simulink library "BBCA_lib"  (Simulink 7.5)
settings: Solver=ode45  StartTime=0.0  StopTime=10.0  RelTol=1e-3
values from neighbouring files (symbols this model uses):
  pBBCA_kPa_VacPresHi_C = Simulink.Parameter    [BBCA_par.m]
  pBBCA_kPa_VacPresLo_C = Simulink.Parameter    [BBCA_par.m]
  pBBCA_pct_PWMOneHundred_C = Simulink.Parameter    [BBCA_par.m]
  pBBCA_pct_PWMZero_C = Simulink.Parameter    [BBCA_par.m]
libraries: BaseOperationLib_Browser x4, simulink x1
settings Model: Creator=wuaibin  LastModifiedBy=wuaibin

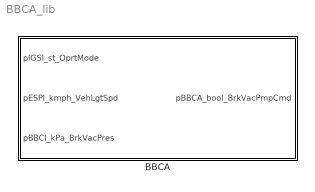
== system BBCA_lib ==
  BBCA : Subsystem  TreatAsAtomicUnit=on

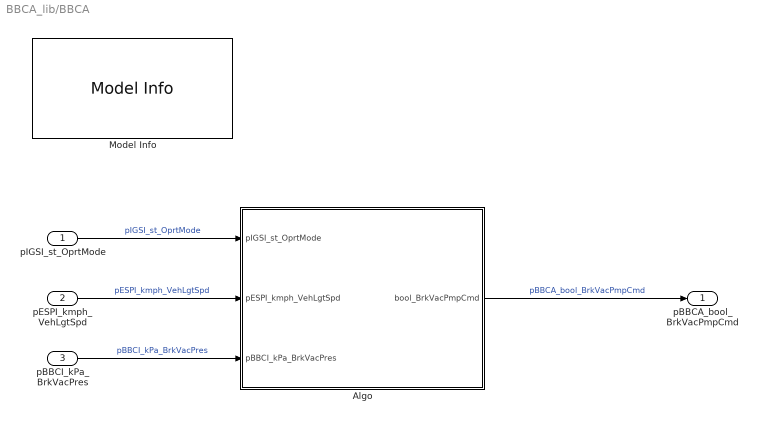
== system BBCA_lib/BBCA ==
  pIGSI_st_OprtMode : Inport  PortDimensions=1  DataType=uint8  OutDataType=fixdt(1, 16)  OutScaling=2^0  OutDataTypeStr=uint8
  pESPI_kmph_VehLgtSpd : Inport  Port=2  PortDimensions=1  DataType=single  OutDataType=fixdt(1, 16)  OutScaling=2^0  OutDataTypeStr=single
  pBBCI_kPa_BrkVacPres : Inport  Port=3  PortDimensions=1  DataType=single  OutDataType=fixdt(1, 16)  OutScaling=2^0  OutDataTypeStr=single
  Algo : Subsystem
  Model Info : simulink/Model-Wide Utilities/Model Info  SystemSampleTime=-1  InitialBlockCM=None  BlockCM=None  Frame=on  DisplayStringWithTags=Model Info\nCreated: %<Created>\nCreator: %<Creator>  HorizontalTextAlignment=Center  LeftAlignmentValue=0.5  SourceBlockDiagram=HQEV_HCU  TagMaxNumber=20
  pBBCA_bool_BrkVacPmpCmd : Outport  OutDataType=fixdt(1, 16)  OutScaling=2^0
  wires:
  Algo/1(bool_BrkVacPmpCmd) -> pBBCA_bool_BrkVacPmpCmd/1  "pBBCA_bool_BrkVacPmpCmd"
  pIGSI_st_OprtMode/1 -> Algo/1(pIGSI_st_OprtMode)  "pIGSI_st_OprtMode"
  pESPI_kmph_VehLgtSpd/1 -> Algo/2(pESPI_kmph_VehLgtSpd)  "pESPI_kmph_VehLgtSpd"
  pBBCI_kPa_BrkVacPres/1 -> Algo/3(pBBCI_kPa_BrkVacPres)  "pBBCI_kPa_BrkVacPres"

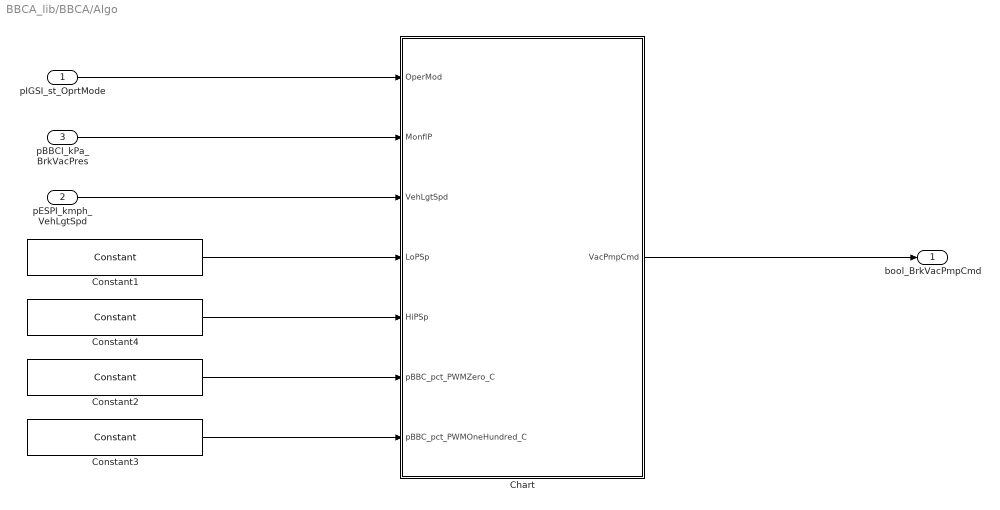
== system BBCA_lib/BBCA/Algo ==
  pIGSI_st_OprtMode : Inport  OutDataType=fixdt(1, 16)  OutScaling=2^0
  pESPI_kmph_VehLgtSpd : Inport  Port=2  OutDataType=fixdt(1, 16)  OutScaling=2^0
  pBBCI_kPa_BrkVacPres : Inport  Port=3  OutDataType=fixdt(1, 16)  OutScaling=2^0
  Chart : Stateflow chart  TreatAsAtomicUnit=on
  Constant1 : BaseOperationLib_Browser/Sources&Sinks/Constant  Value=pBBCA_kPa_VacPresLo_C  OutMin=[]  OutMax=[]  OutDataType=fixdt(1, 16)  ConRadixGroup=Use specified scaling  OutScaling=2^0  OutDataTypeStr=Inherit: Inherit from 'Constant value'
  Constant2 : BaseOperationLib_Browser/Sources&Sinks/Constant  Value=pBBCA_pct_PWMZero_C  OutMin=[]  OutMax=[]  OutDataType=fixdt(1, 16)  ConRadixGroup=Use specified scaling  OutScaling=2^0  OutDataTypeStr=Inherit: Inherit from 'Constant value'
  Constant3 : BaseOperationLib_Browser/Sources&Sinks/Constant  Value=pBBCA_pct_PWMOneHundred_C  OutMin=[]  OutMax=[]  OutDataType=fixdt(1, 16)  ConRadixGroup=Use specified scaling  OutScaling=2^0  OutDataTypeStr=Inherit: Inherit from 'Constant value'
  Constant4 : BaseOperationLib_Browser/Sources&Sinks/Constant  Value=pBBCA_kPa_VacPresHi_C  OutMin=[]  OutMax=[]  OutDataType=fixdt(1, 16)  ConRadixGroup=Use specified scaling  OutScaling=2^0  OutDataTypeStr=Inherit: Inherit from 'Constant value'
  bool_BrkVacPmpCmd : Outport  OutDataType=fixdt(1, 16)  OutScaling=2^0
  wires:
  Constant4/1 -> Chart/5(HiPSp)
  Constant1/1 -> Chart/4(LoPSp)
  pESPI_kmph_VehLgtSpd/1 -> Chart/3(VehLgtSpd)
  pIGSI_st_OprtMode/1 -> Chart/1(OperMod)
  pBBCI_kPa_BrkVacPres/1 -> Chart/2(MonflP)
  Chart/1(VacPmpCmd) -> bool_BrkVacPmpCmd/1
  Constant2/1 -> Chart/6(pBBC_pct_PWMZero_C)
  Constant3/1 -> Chart/7(pBBC_pct_PWMOneHundred_C)

== stateflow chart BBCA/Algo/Chart ==
  state PmpOff
    entry:
    VacPmpCmd = pBBC_pct_PWMZero_C;
  state PmpOn
    en:
    VacPmpCmd = pBBC_pct_PWMOneHundred_C;
  (default) -> PmpOff
  PmpOff -> PmpOn : [(OperMod >= OperModTyp.CL15 || VehLgtSpd > p_BBC_VehLgtSpdThd_kmph)...
      | && (MonflP >= LoPSp)]
  PmpOn -> PmpOff : [(OperMod == OperModTyp.IG_OFF && VehLgtSpd < p_BBC_VehLgtSpdThd_kmph)...
      | || (MonflP <= HiPSp)]
  data: OperMod input double; MonflP input double; VacPmpCmd output uint8; VehLgtSpd input double; LoPSp input double; HiPSp input double; p_BBC_VehLgtSpdThd_kmph parameter double; pBBC_pct_PWMZero_C input double; pBBC_pct_PWMOneHundred_C input double
